simulink model "RR_Robot_kin"  (R2019a)
settings: Solver=VariableStepAuto  StartTime=0.0  StopTime=5  RelTol=1e-3
values from neighbouring files (symbols this model uses):
  l1 = 1    [forwardKinematics.m]    (also in inverseKinematics.m)
  l2 = 1    [forwardKinematics.m]    (also in inverseKinematics.m)
libraries: mblibv1 x11, simulink x2
settings Model: Creator=Shashank  LastModifiedBy=Shashank

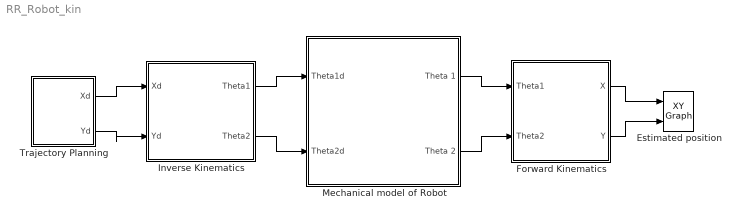
== system RR_Robot_kin ==
  Estimated position : simulink/Sinks/XY Graph  xmin=0.5  xmax=1.5  ymin=0.5  ymax=1.5  st=-1
  Forward Kinematics : MATLAB Function  TreatAsAtomicUnit=on
  Inverse Kinematics : MATLAB Function  TreatAsAtomicUnit=on
  Mechanical model of Robot : Subsystem
  Trajectory Planning : Subsystem
  wires:
  Forward Kinematics/1(X) -> Estimated position/1
  Forward Kinematics/2(Y) -> Estimated position/2
  Inverse Kinematics/1(Theta1) -> Mechanical model of Robot/1(Theta1d)
  Inverse Kinematics/2(Theta2) -> Mechanical model of Robot/2(Theta2d)
  Mechanical model of Robot/1(Theta 1) -> Forward Kinematics/1(Theta1)
  Mechanical model of Robot/2(Theta 2) -> Forward Kinematics/2(Theta2)
  Trajectory Planning/1(Xd) -> Inverse Kinematics/1(Xd)
  Trajectory Planning/2(Yd) -> Inverse Kinematics/2(Yd)

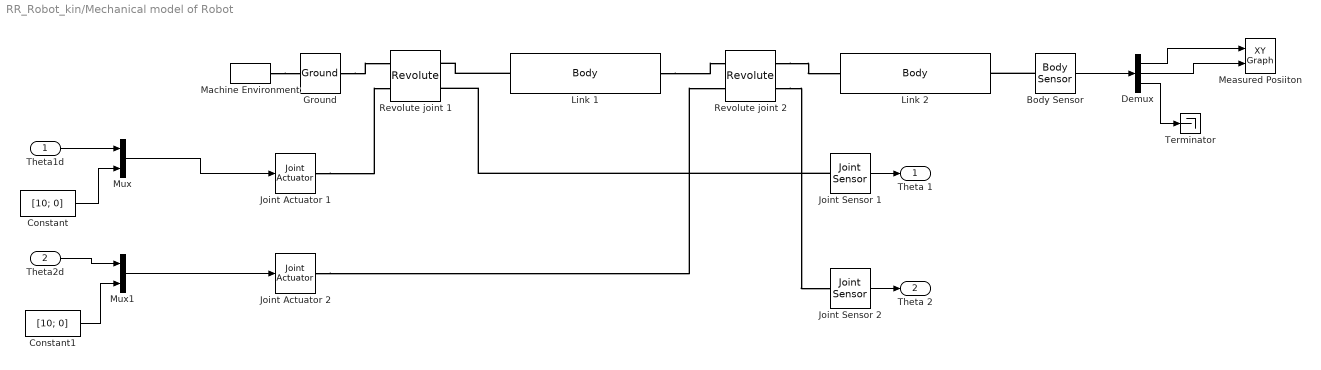
== system RR_Robot_kin/Mechanical model of Robot ==
  Theta1d : Inport
  Theta2d : Inport  Port=2
  Body Sensor : mblibv1/Sensors &  Actuators/Body Sensor  UpdateFromCAD=off  PhysicalDomain=Mechanical  PortType=blob  Muxed=on  Pose=off  Angle=on  AngleUnits=deg  ArcVelocity=off  ArcVelocityUnits=deg/s  ArcAcceleration=off  ArcAccelerationUnits=deg/s^2  CoordPosition=on  CoordPositionUnits=m  Velocity=off  VelocityUnits=m/s  Acceleration=off  AccelerationUnits=m/s^2  Quaternion=on  QuaternionDT=off  QuaternionDDT=off  QuaternionUnits=off  OutputVector=[1]  ActiveIO=on  Width=3  DialogClass=MechanicalSensorBlock  ReferenceFrame=Absolute (World)
      settings: SourceProductName=Simscape Multibody  SourceProductBaseCode=MS
  Constant : Constant  Value=[10; 0]
  Constant1 : Constant  Value=[10; 0]
  Demux : Demux  Outputs=3
  Ground : mblibv1/Bodies/Ground  UpdateFromCAD=off  LeftPortType=env  RightPortType=workingframe  PhysicalDomain=Mechanical  DialogClass=GroundBlock  CoordPosition=[0 0 0]  CoordPositionUnits=m  StateVectorMgrId=0  MachineId=[1 0]  ShowEnvPort=on  ParameterChecksum=[3991527807, 2032448827, 3448428237, 557945592]  TopologyChecksum=[956111145, 1829508211, 3573501221, 755807185]
      settings: SourceProductName=Simscape Multibody  SourceProductBaseCode=MS
  Joint Actuator 1 : mblibv1/Sensors &  Actuators/Joint Actuator  UpdateFromCAD=off  PhysicalDomain=Mechanical  PortType=blob  ActuationStyle=Motion  AngleUnits=rad  ArcVelocityUnits=rad/s  ArcAccelerationUnits=rad/s^2  CoordPositionUnits=m  VelocityUnits=m/s  AccelerationUnits=m/s^2  ForceUnits=N  TorqueUnits=N*m  ActiveIO=on  Width=3  DialogClass=MechanicalActuatorBlock  Primitive=R1  ReferenceFrame=Absolute (World)
      settings: SourceProductName=Simscape Multibody  SourceProductBaseCode=MS
  Joint Actuator 2 : mblibv1/Sensors &  Actuators/Joint Actuator  UpdateFromCAD=off  PhysicalDomain=Mechanical  PortType=blob  ActuationStyle=Motion  AngleUnits=rad  ArcVelocityUnits=rad/s  ArcAccelerationUnits=rad/s^2  CoordPositionUnits=m  VelocityUnits=m/s  AccelerationUnits=m/s^2  ForceUnits=N  TorqueUnits=N*m  ActiveIO=on  Width=3  DialogClass=MechanicalActuatorBlock  Primitive=R1  ReferenceFrame=Absolute (World)
      settings: SourceProductName=Simscape Multibody  SourceProductBaseCode=MS
  "Joint Sensor 1 " : mblibv1/Sensors &  Actuators/Joint Sensor  UpdateFromCAD=off  PhysicalDomain=Mechanical  PortType=blob  Muxed=on  Pose=off  Angle=on  AngleUnits=rad  ArcVelocity=off  ArcVelocityUnits=deg/s  ArcAcceleration=off  ArcAccelerationUnits=deg/s^2  CoordPosition=on  CoordPositionUnits=m  Velocity=off  VelocityUnits=m/s  Acceleration=off  AccelerationUnits=m/s^2  Quaternion=on  QuaternionDT=off  QuaternionDDT=off  QuaternionUnits=off  OutputVector=[1]  ActiveIO=on  Width=1  DialogClass=MechanicalSensorBlock  Primitive=R1  Force=off  ForceUnits=N  Torque=off  TorqueUnits=N*m  ReferenceFrame=Absolute (World)  ReactionSensedSide=Base  ReactionReferenceFrame=Absolute (World)  ReactionForce=off  ReactionForceUnits=N  ReactionMoment=off  ReactionMomentUnits=N*m
      settings: SourceProductName=Simscape Multibody  SourceProductBaseCode=MS
  Joint Sensor 2 : mblibv1/Sensors &  Actuators/Joint Sensor  UpdateFromCAD=off  PhysicalDomain=Mechanical  PortType=blob  Muxed=on  Pose=off  Angle=on  AngleUnits=rad  ArcVelocity=off  ArcVelocityUnits=deg/s  ArcAcceleration=off  ArcAccelerationUnits=deg/s^2  CoordPosition=on  CoordPositionUnits=m  Velocity=off  VelocityUnits=m/s  Acceleration=off  AccelerationUnits=m/s^2  Quaternion=on  QuaternionDT=off  QuaternionDDT=off  QuaternionUnits=off  OutputVector=[1]  ActiveIO=on  Width=1  DialogClass=MechanicalSensorBlock  Primitive=R1  Force=off  ForceUnits=N  Torque=off  TorqueUnits=N*m  ReferenceFrame=Absolute (World)  ReactionSensedSide=Base  ReactionReferenceFrame=Absolute (World)  ReactionForce=off  ReactionForceUnits=N  ReactionMoment=off  ReactionMomentUnits=N*m
      settings: SourceProductName=Simscape Multibody  SourceProductBaseCode=MS
  Link 1 : mblibv1/Bodies/Body  LConnTagsString=CS1  RConnTagsString=CS2  UpdateFromCAD=off  DialogClass=MechanicalBodyBlock  Mass=1  MassUnits=kg  InertiaUnits=kg*m^2  Inertia=eye(3)  Shape=Cylinder  ShapeDims=[1 1]  ShapeUnits=m  ShapeUse=false  Density=1  DensityUnits=kg/m^3  DensityUse=false  GraphicsMode=MACHINE_DEFAULT  BodyColorSelMode=MACHINE_DEFAULT  BodyColor=[1 0 0]  AttachedToCS=CG  CG=Left$CG$[0 0 0]$WORLD$WORLD$m$[0 0 0]$Euler X-Y-Z$deg$WORLD$false$none  WorkingFrames=Left$CS1$[0 0 0]$World$World$m$[0 0 0]$Euler X-Y-Z$deg$WORLD$true$none#Right$CS2$[l1 0 0]$CG$CG$m$[0 0 0]$Euler X-Y-Z$deg$WORLD$true$none  CGPos=[0 0 0]  CGRot=[0 0 0]  CS0Pos=[]  CS0Rot=[]  CS1Pos=[0 0 0]  CS1Rot=[0 0 0]  CS2Pos=[l1 0 0]  CS2Rot=[0 0 0]  CS3Pos=[]  CS3Rot=[]  CS4Pos=[]  CS4Rot=[]  CS5Pos=[]  CS5Rot=[]  CS6Pos=[]  CS6Rot=[]  CS7Pos=[]  CS7Rot=[]  CS8Pos=[]  CS8Rot=[]  CS9Pos=[]  CS9Rot=[]  CS10Pos=[]  CS10Rot=[]  CS11Pos=[]  CS11Rot=[]  CS12Pos=[]  CS12Rot=[]  CS13Pos=[]  CS13Rot=[]  CS14Pos=[]  CS14Rot=[]  CS15Pos=[]  CS15Rot=[]  CS16Pos=[]  CS16Rot=[]  CS17Pos=[]  CS17Rot=[]  CS18Pos=[]  CS18Rot=[]  CS19Pos=[]  CS19Rot=[]  CS20Pos=[]  CS20Rot=[]
      settings: SourceProductName=Simscape Multibody  SourceProductBaseCode=MS
  Link 2 : mblibv1/Bodies/Body  LConnTagsString=CS1  RConnTagsString=CS2  UpdateFromCAD=off  DialogClass=MechanicalBodyBlock  Mass=1  MassUnits=kg  InertiaUnits=kg*m^2  Inertia=eye(3)  Shape=Cylinder  ShapeDims=[1 1]  ShapeUnits=m  ShapeUse=false  Density=1  DensityUnits=kg/m^3  DensityUse=false  GraphicsMode=MACHINE_DEFAULT  BodyColorSelMode=MACHINE_DEFAULT  BodyColor=[1 0 0]  AttachedToCS=CG  CG=Left$CG$[0 0 0]$WORLD$WORLD$m$[0 0 0]$Euler X-Y-Z$deg$WORLD$false$none  WorkingFrames=Left$CS1$[0 0 0]$Adjoining$Adjoining$m$[0 0 0]$Euler X-Y-Z$deg$WORLD$true$none#Right$CS2$[l2 0 0]$CS1$CS1$m$[0 0 0]$Euler X-Y-Z$deg$WORLD$true$none  CGPos=[0 0 0]  CGRot=[0 0 0]  CS0Pos=[]  CS0Rot=[]  CS1Pos=[0 0 0]  CS1Rot=[0 0 0]  CS2Pos=[l2 0 0]  CS2Rot=[0 0 0]  CS3Pos=[]  CS3Rot=[]  CS4Pos=[]  CS4Rot=[]  CS5Pos=[]  CS5Rot=[]  CS6Pos=[]  CS6Rot=[]  CS7Pos=[]  CS7Rot=[]  CS8Pos=[]  CS8Rot=[]  CS9Pos=[]  CS9Rot=[]  CS10Pos=[]  CS10Rot=[]  CS11Pos=[]  CS11Rot=[]  CS12Pos=[]  CS12Rot=[]  CS13Pos=[]  CS13Rot=[]  CS14Pos=[]  CS14Rot=[]  CS15Pos=[]  CS15Rot=[]  CS16Pos=[]  CS16Rot=[]  CS17Pos=[]  CS17Rot=[]  CS18Pos=[]  CS18Rot=[]  CS19Pos=[]  CS19Rot=[]  CS20Pos=[]  CS20Rot=[]
      settings: SourceProductName=Simscape Multibody  SourceProductBaseCode=MS
  Machine Environment : mblibv1/Bodies/Machine Environment  PortType=env  PhysicalDomain=Mechanical  DialogTemplateClass=MECH.MachineEnvironment  SyncWhenCopied=off  Gravity=[0 -9.81 0]  GravityUnits=m/s^2  GravityAsSignal=off  Dimensionality=Auto-detect  AnalysisType=Forward dynamics  LinearAssemblyTolerance=1e-3  LinearAssemblyToleranceUnits=m  AngularAssemblyTolerance=1e-3  AngularAssemblyToleranceUnits=rad  ConstraintSolverType=Stabilizing  ConstraintRelTolerance=1e-4  ConstraintAbsTolerance=1e-4  UseRobustSingularityHandling=off  RedundancyAnalysisToleranceType=Automatically select tolerance  RedundancyAnalysisTolerance=1e-14  StatePerturbationType=Fixed  PerturbationSize=1e-5  VisualizeMachine=on  BodyVisualizationType=Use model default body geometries  BodyColorSelMode=Use model default  DefaultBodyColor=[1 0 0]
      settings: SourceProductName=Simscape Multibody  SourceProductBaseCode=MS
  Measured Posiiton : simulink/Sinks/XY Graph  xmin=0.5  xmax=1.5  ymin=0.5  ymax=1.5  st=-1
  Mux : Mux  Inputs=2
  Mux1 : Mux  Inputs=2
  Revolute joint 1 : mblibv1/Joints/Revolute  LConnTagsString=__newl0|SA1  RConnTagsString=__newr0|SA1  UpdateFromCAD=off  NumSAPorts=2  CutJoint=off  MarkAsCut=off  Primitives=prismatic  PrimitiveProps=R1$World$[0 0 1]$revolute  DialogClass=JointBlock  R1Axis=[0 0 1]
      settings: SourceProductName=Simscape Multibody  SourceProductBaseCode=MS
  Revolute joint 2 : mblibv1/Joints/Revolute  LConnTagsString=__newl0|SA1  RConnTagsString=__newr0|SA1  UpdateFromCAD=off  NumSAPorts=2  CutJoint=off  MarkAsCut=off  Primitives=prismatic  PrimitiveProps=R1$World$[0 0 1]$revolute  DialogClass=JointBlock  R1Axis=[0 0 1]
      settings: SourceProductName=Simscape Multibody  SourceProductBaseCode=MS
  Terminator : Terminator
  Theta 1 : Outport
  Theta 2 : Outport  Port=2
  wires:
  "Joint Sensor 1 "/1 -> Theta 1/1
  Body Sensor/1 -> Demux/1
  Demux/2 -> Measured Posiiton/2
  Theta2d/1 -> Mux1/1
  Demux/3 -> Terminator/1
  Demux/1 -> Measured Posiiton/1
  Theta1d/1 -> Mux/1
  Constant/1 -> Mux/2
  Constant1/1 -> Mux1/2
  Mux1/1 -> Joint Actuator 2/1
  Mux/1 -> Joint Actuator 1/1
  Joint Sensor 2/1 -> Theta 2/1
  connections:
  "Joint Sensor 1 "/LConn1 -- Revolute joint 1/RConn2
  Ground/RConn1 -- Revolute joint 1/LConn1
  Joint Actuator 1/RConn1 -- Revolute joint 1/LConn2
  Body Sensor/LConn1 -- Link 2/RConn1
  Revolute joint 2/RConn2 -- Joint Sensor 2/LConn1
  Link 1/RConn1 -- Revolute joint 2/LConn1
  Machine Environment/RConn1 -- Ground/LConn1
  Link 1/LConn1 -- Revolute joint 1/RConn1
  Joint Actuator 2/RConn1 -- Revolute joint 2/LConn2
  Revolute joint 2/RConn1 -- Link 2/LConn1

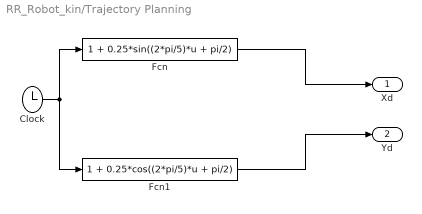
== system RR_Robot_kin/Trajectory Planning ==
  Clock : Clock
  Fcn : Fcn  Expr=1 + 0.25*sin((2*pi/5)*u + pi/2)
  Fcn1 : Fcn  Expr=1 + 0.25*cos((2*pi/5)*u + pi/2)
  Xd : Outport
  Yd : Outport  Port=2
  wires:
  Clock/1 -> Fcn1/1, Fcn/1
  Fcn/1 -> Xd/1
  Fcn1/1 -> Yd/1

== matlab function RR_Robot_kin/Inverse Kinematics ==
  data: Xd input; Theta1 output; Yd input; Theta2 output
function [Theta1,Theta2] = InverseKinematics(Xd,Yd)

l1 = 1;
l2 = 1;

Theta2 = acos((Xd^2+Yd^2 - l1^2 - l2^2)/(2*l1*l2));

s_Theta2 = sin(Theta2);
c_Theta2 = cos(Theta2);

Theta1 = atan2(Yd,Xd) - atan2(l2*s_Theta2, (l1+l2*c_Theta2));

== matlab function RR_Robot_kin/Forward Kinematics ==
  data: Theta1 input; X output; Theta2 input; Y output
function [X,Y] = Forwardkinematics(Theta1, Theta2)

l1 = 1;
l2 = 1;

T10 = [cos(Theta1), -sin(Theta1), 0, l1*cos(Theta1);
    sin(Theta1), cos(Theta1), 0, l1*sin(Theta1);
    0, 0, 1, 0;
    0, 0, 0, 1];

T21 = [cos(Theta2), -sin(Theta2), 0, l1*cos(Theta2);
    sin(Theta2), cos(Theta2), 0, l1*sin(Theta2);
    0, 0, 1, 0;
    0, 0, 0, 1];

T20 = T10*T21;

X = T20(1,4);
Y = T20(2,4);
